simulink model "lab_03_something"  (R2024b)
settings: Solver=VariableStepAuto  StartTime=0.0  StopTime=10.0  RelTol=1e-3

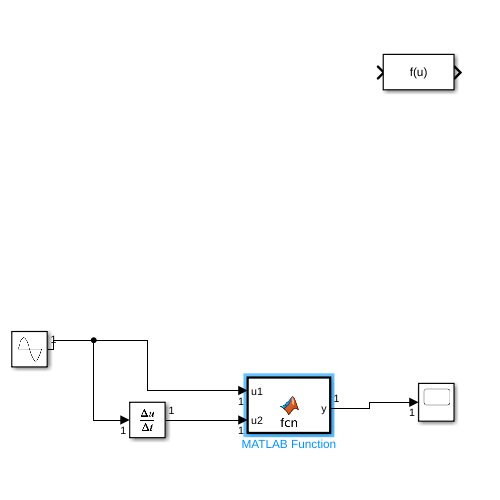
[thumbnail: Simulink's stored preview of the top-level diagram]
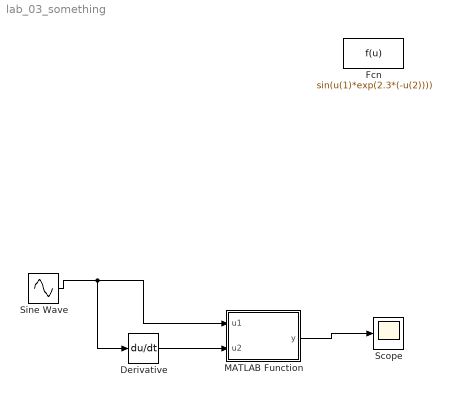
== system lab_03_something ==
  Derivative : Derivative
  Fcn : Fcn  Expr=sin(u(1)*exp(2.3*(-u(2))))
  MATLAB Function : MATLAB Function  TreatAsAtomicUnit=on
  Scope : Scope
  Sine Wave : Sin  SampleTime=0
  wires:
  Sine Wave/1 -> Derivative/1, MATLAB Function/1(u1)
  Derivative/1 -> MATLAB Function/2(u2)
  MATLAB Function/1(y) -> Scope/1

== matlab function lab_03_something/MATLAB Function ==
  data: u1 input; y output; u2 input
function y = fcn(u1,u2)

y = conv(u1,u2);
